simulink subsystem "ElectricalThermalSystemSSC"  (R2025a)
settings: Solver=VariableStepAuto  StartTime=0.0  StopTime=10.0  RelTol=1e-3
undefined symbols (not defined in the file): coolant_pipe_D, coolant_valve_D_ratio_max, coolant_valve_D_ratio_min, coolant_valve_displacement, EnvAirTemp, EnvGrvty, PlantThrEstCmpPwr, PlntThrChArea, PlntThrFanMaxSpd, PlntThrFanMechEff, PlntThrFanVolEff, PlntThrHeaterMaxPwr, PlntThrPipeArea, PlntThrPipeDia, PlntThrPmpMaxSpd, PlntThrRadRamEff, PlntThrRefrigAinit, PlntThrTankArea, PlntThrTankVol, PlntThrValDisp, PlntThrValDratioMax, PlntThrValDratioMin, PlntThrValSplMax, ThrmEM1, ThrmEM2, ThrmEM3, ThrmEM4
libraries: fl_lib x159, nesl_utility x69, SimscapeFluids_lib x25, autolibutils x12
(part 1 of 5)
settings Model: ModifiedByFormat=The MathWorks, Inc.  Creator=The MathWorks, Inc.  LastModifiedBy=The MathWorks, Inc.
settings SolverCC: MaxZcPerStep=1.0
settings OptimizationCC: ReuseModelBlockBuffer=off
settings DebuggingCC: UnconnectedInputMsg=warning  UnconnectedOutputMsg=warning  UnconnectedLineMsg=warning  SubsystemReferenceDiagnosticForUnitTest=warning
settings ModelReferenceCC: EnableRefExpFcnMdlSchedulingChecks=on
settings RTWCC: GPUComputeCapability=3.5  DLArmComputeVersion=19.05  LargeConstantGeneration=WriteOnlyDNNConstantsToDataFiles
settings CodeAppCC: StateflowObjectComments=on

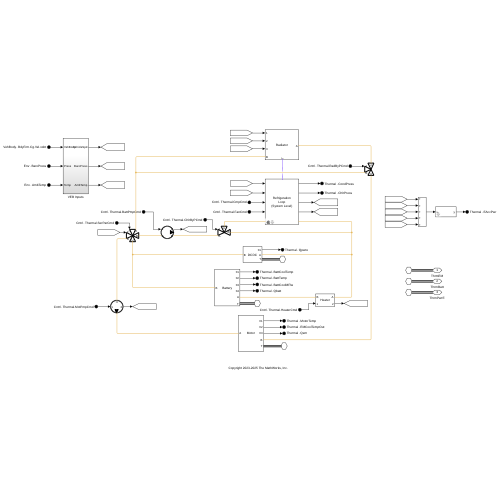
[thumbnail: Simulink's stored preview of the top-level diagram]
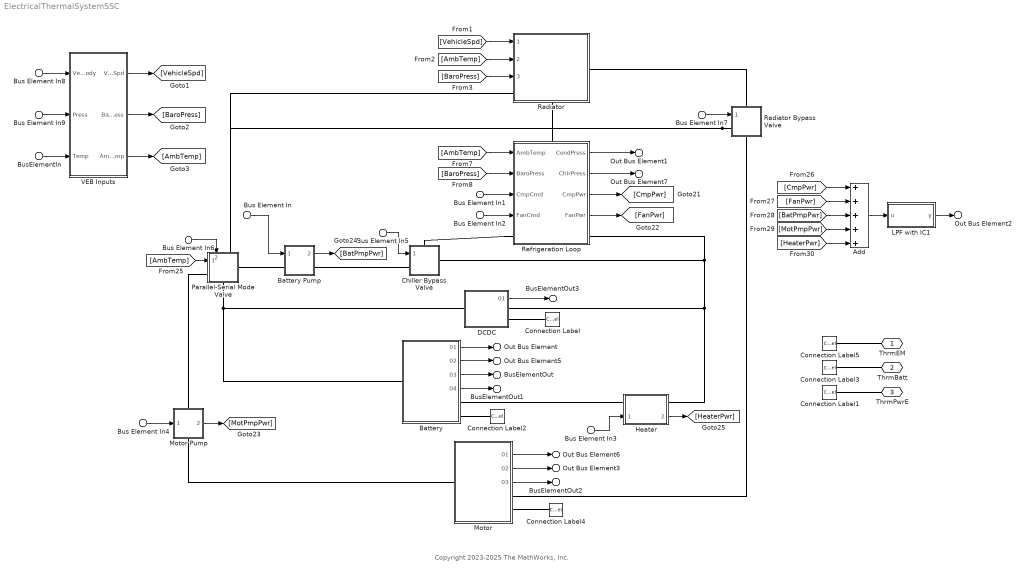
== system ElectricalThermalSystemSSC ==
  note: Copyright 2023-2025 The MathWorks, Inc.
  Bus Element In4 : Inport  PortName=Cntrl  Element=Thermal.MotPmpCmd
  Bus Element In6 : Inport  PortName=Cntrl  Element=Thermal.SerParCmd
  Bus Element In2 : Inport  PortName=Cntrl  Element=Thermal.FanCmd
  Bus Element In7 : Inport  PortName=Cntrl  Element=Thermal.RadByPCmd
  Bus Element In1 : Inport  PortName=Cntrl  Element=Thermal.CmpCmd
  Bus Element In3 : Inport  PortName=Cntrl  Element=Thermal.HeaterCmd
  Bus Element In : Inport  PortName=Cntrl  Element=Thermal.BattPmpCmd
  Bus Element In5 : Inport  PortName=Cntrl  Element=Thermal.ChlrByPCmd
  Bus Element In8 : Inport  Port=2  PortName=VehBody  Element=BdyFrm.Cg.Vel.xdot
  Bus Element In9 : Inport  Port=3  PortName=Env  Element=BaroPress
  BusElementIn : Inport  Port=3  PortName=Env  Element=AmbTemp
  Add : Sum  Inputs=+++++
  Battery : Subsystem  Tag=PublishSubsystem
      mask Display: disp(get_param(gcb, 'Name'))
  Battery Pump : Subsystem  Tag=PublishSubsystem
      mask Display:
      | plot(100*cos(linspace(0, 2*pi, 500)), 100*sin(linspace(0, 2*pi, 500)))
      | patch([100 55 55 100]-1, [0 24 -24 0], [0 0 0])
  Chiller Bypass Valve : Subsystem  Tag=PublishSubsystem
      settings: PortSchema="{\"entries\":[{\"content\":{\"sides\":[{\"content\":{\"connectorIds\":[\"In1\",\"LConn1\"]},\"type\":\"ConnectorPlacement.EquallySpacedRectSide\",\"uuid\":\"6d832dc2-b60e-40b1-a4f2-705eabcb1b94\"},{\"content\":{\"connectorIds\":[\"RConn1\"],\"side\":\"RIGHT\"},\"type\":\"ConnectorPlacement.EquallySpacedRectSide\",\"uuid\":\"14466d4b-d366-4217-9b68-7dedef557cda\"},{\"content\":{\"connectorIds\":[\"LConn2\"],\"side\":\"TOP\"},\"type\":\"ConnectorPlacement.EquallySpacedRectSide\",\"uuid\":\"a673b71e-6232-4949-9217-0d4d0fced751\"}]},\"type\":\"ConnectorPlacement.EquallySpacedConnector\",\"uuid\":\"e7c23af8-b365-4139-b104-c2b6ff749898\"}],\"packageUris\":[\"http://schema.mathworks.com/mf0/Connector/R2020b\"],\"version\":\"1.0\"}"
      mask Display:
      | color('white')
      | plot(100, 100)
      | plot(-100, -100)
      | color('black')
      | 
      | plot([0 -100 -100 0], [0 50 -50 0])
      | plot([0 100 100 0], [0 50 -50 0])
      | plot([0 50 -50 0], [0 100 100 0])
  Connection Label : ConnectionLabel  Label=ThrmPwrE
  Connection Label1 : ConnectionLabel  Label=ThrmPwrE
  Connection Label2 : ConnectionLabel  Label=ThrmBatt
  Connection Label3 : ConnectionLabel  Label=ThrmBatt
  Connection Label4 : ConnectionLabel  Label=ThrmEM
  Connection Label5 : ConnectionLabel  Label=ThrmEM
  DCDC : Subsystem  Tag=PublishSubsystem
      mask Display: disp(get_param(gcb, 'Name'))
  Heater : Subsystem  Tag=PublishSubsystem
      mask Display: disp(get_param(gcb, 'Name'))
  LPF with IC1 : Subsystem  mask{wc=10, InitCond=0, dataType=off}
      mask prompts: wc "Cutoff frequency, wc [rad/s]"; InitCond "Initial condition, InitCond [same as u]"; dataType "Enforce same input data type"
      mask TypeOptions wc: Cont LPF IC/wc
      mask TypeOptions InitCond: Initial Condition/Value
      mask TypeOptions dataType: Cont LPF IC/dataType
  Motor : Subsystem  Tag=PublishSubsystem
      mask Display: disp(get_param(gcb, 'Name'))
  Motor Pump : Subsystem  Tag=PublishSubsystem
      settings: PortSchema="{\"entries\":[{\"content\":{\"sides\":[{\"content\":{\"connectorIds\":[\"In1\"]},\"type\":\"ConnectorPlacement.EquallySpacedRectSide\",\"uuid\":\"998a9c6b-bb40-4bcc-a380-2cd5a078b990\"},{\"content\":{\"connectorIds\":[\"Out1\"],\"side\":\"RIGHT\"},\"type\":\"ConnectorPlacement.EquallySpacedRectSide\",\"uuid\":\"42ec83ef-b217-4586-a8aa-6044af8db7a9\"},{\"content\":{\"connectorIds\":[\"LConn1\"],\"side\":\"TOP\"},\"type\":\"ConnectorPlacement.EquallySpacedRectSide\",\"uuid\":\"eeac28b9-ebf8-455e-ab0a-fa40d1d96b1a\"},{\"content\":{\"connectorIds\":[\"RConn1\"],\"side\":\"BOTTOM\"},\"type\":\"ConnectorPlacement.EquallySpacedRectSide\",\"uuid\":\"020a4ae5-c25e-4792-8687-aa24bac3421e\"}]},\"type\":\"ConnectorPlacement.EquallySpacedConnector\",\"uuid\":\"d6a5444d-a0f8-4af1-be22-0f458325ee39\"}],\"packageUris\":[\"http://schema.mathworks.com/mf0/Connector/R2020b\"],\"version\":\"1.0\"}"
      mask Display:
      | plot(100*cos(linspace(0, 2*pi, 500)), 100*sin(linspace(0, 2*pi, 500)))
      | patch([0 24 -24 0], [-100 -55 -55 -100]+1, [0 0 0])
  Parallel-Serial Mode Valve : Subsystem  Tag=PublishSubsystem
      settings: PortSchema="{\"entries\":[{\"content\":{\"sides\":[{\"content\":{\"connectorIds\":[\"In1\",\"LConn1\"]},\"type\":\"ConnectorPlacement.EquallySpacedRectSide\",\"uuid\":\"0e85f4fb-5a75-439f-b35d-71055581b22a\"},{\"content\":{\"connectorIds\":[\"RConn1\"],\"side\":\"RIGHT\"},\"type\":\"ConnectorPlacement.EquallySpacedRectSide\",\"uuid\":\"a94d9cc9-a388-4b39-8755-f80106b7cded\"},{\"content\":{\"connectorIds\":[\"In2\",\"LConn2\"],\"side\":\"TOP\"},\"type\":\"ConnectorPlacement.EquallySpacedRectSide\",\"uuid\":\"13934e59-9fe7-4603-811a-b738b7f2468b\"},{\"content\":{\"connectorIds\":[\"RConn2\"],\"side\":\"BOTTOM\"},\"type\":\"ConnectorPlacement.EquallySpacedRectSide\",\"uuid\":\"987fbf53-7ea1-4dfb-bf26-1dc5077683a8\"}]},\"type\":\"ConnectorPlacement.EquallySpacedConnector\",\"uuid\":\"a78c426f-33db-4869-ab6d-8416109da949\"}],\"packageUris\":[\"http://schema.mathworks.com/mf0/Connector/R2020b\"],\"version\":\"1.0\"}"
      mask Display:
      | color('white')
      | plot(100, 100)
      | plot(-100, -100)
      | color('black')
      | 
      | plot([0 -100 -100 0], [0 50 -50 0])
      | plot([0 100 100 0], [0 50 -50 0])
      | plot([0 50 -50 0], [0 100 100 0])
      | plot([0 50 -50 0], [0 -100 -100 0])
  Radiator : Subsystem  Tag=PublishSubsystem
      settings: PortSchema="{\"entries\":[{\"content\":{\"sides\":[{\"content\":{\"connectorIds\":[\"In1\",\"In2\",\"In3\",\"LConn1\"]},\"type\":\"ConnectorPlacement.EquallySpacedRectSide\",\"uuid\":\"99a54269-bbf6-4ded-87b9-61a0201744d3\"},{\"content\":{\"connectorIds\":[\"RConn1\"],\"side\":\"RIGHT\"},\"type\":\"ConnectorPlacement.EquallySpacedRectSide\",\"uuid\":\"97272aa5-cf38-4f1e-876b-ad8adb9bd6e5\"},{\"content\":{\"side\":\"TOP\"},\"type\":\"ConnectorPlacement.EquallySpacedRectSide\",\"uuid\":\"c8198971-aa26-402f-9339-3fbe814dbf96\"},{\"content\":{\"connectorIds\":[\"RConn2\"],\"side\":\"BOTTOM\"},\"type\":\"ConnectorPlacement.EquallySpacedRectSide\",\"uuid\":\"78457e8c-40ee-463d-bbac-3ff68067e992\"}]},\"type\":\"ConnectorPlacement.EquallySpacedConnector\",\"uuid\":\"b91fbaf9-058c-42a3-b093-b88166909bf7\"}],\"packageUris\":[\"http://schema.mathworks.com/mf0/Connector/R2020b\"],\"version\":\"1.0\"}"
      mask Display: disp(get_param(gcb, 'Name'))
  Radiator Bypass Valve : Subsystem  Tag=PublishSubsystem
      settings: PortSchema="{\"entries\":[{\"content\":{\"sides\":[{\"content\":{\"connectorIds\":[\"In1\",\"LConn1\"]},\"type\":\"ConnectorPlacement.EquallySpacedRectSide\",\"uuid\":\"098431ba-fd37-427d-ab99-1fdc173a8d83\"},{\"content\":{\"side\":\"RIGHT\"},\"type\":\"ConnectorPlacement.EquallySpacedRectSide\",\"uuid\":\"bb877428-37aa-42a4-9b6a-b528d13b970d\"},{\"content\":{\"connectorIds\":[\"LConn2\"],\"side\":\"TOP\"},\"type\":\"ConnectorPlacement.EquallySpacedRectSide\",\"uuid\":\"3621d48a-02c0-4e61-a0fa-118fe0650d0a\"},{\"content\":{\"connectorIds\":[\"RConn1\"],\"side\":\"BOTTOM\"},\"type\":\"ConnectorPlacement.EquallySpacedRectSide\",\"uuid\":\"1f4bac76-5544-4b75-8f5a-621b64243fb7\"}]},\"type\":\"ConnectorPlacement.EquallySpacedConnector\",\"uuid\":\"706d2219-b4aa-4013-bee1-17248f8b2a38\"}],\"packageUris\":[\"http://schema.mathworks.com/mf0/Connector/R2020b\"],\"version\":\"1.0\"}"
      mask Display:
      | color('white')
      | plot(100, 100)
      | plot(-100, -100)
      | color('black')
      | 
      | plot([0 -100 -100 0], [0 50 -50 0])
      | plot([0 50 -50 0], [0 100 100 0])
      | plot([0 50 -50 0], [0 -100 -100 0])
  Refrigeration Loop : Subsystem  Tag=detailed cycle  Variant=on  VariantControlMode=label  VariantControl=Choice  LabelModeActiveChoice=System Level  mask{SystemChoice=System Level}
      mask prompts: SystemChoice "Choose a variant:"
      settings: PortSchema="{\"entries\":[{\"content\":{\"sides\":[{\"content\":{\"connectorIds\":[\"In1\",\"In2\",\"In3\",\"In4\",\"LConn1\"]},\"type\":\"ConnectorPlacement.EquallySpacedRectSide\",\"uuid\":\"4e244fff-03f9-4340-b01c-d55ca64bfb01\"},{\"content\":{\"connectorIds\":[\"Out1\",\"Out2\",\"Out3\",\"Out4\",\"RConn1\"],\"side\":\"RIGHT\"},\"type\":\"ConnectorPlacement.EquallySpacedRectSide\",\"uuid\":\"d8829212-1983-4dc7-b137-b6bce8b26069\"},{\"content\":{\"connectorIds\":[\"LConn2\"],\"side\":\"TOP\"},\"type\":\"ConnectorPlacement.EquallySpacedRectSide\",\"uuid\":\"473d2e24-2387-478c-ae11-a4bbaffe09fe\"}]},\"type\":\"ConnectorPlacement.EquallySpacedConnector\",\"uuid\":\"f4265e97-c303-48ef-b1e0-f8b1ed3e0934\"}],\"packageUris\":[\"http://schema.mathworks.com/mf0/Connector/R2020b\"],\"version\":\"1.0\"}"
      mask TypeOptions SystemChoice: System Level | Power Estimate
      mask Callback SystemChoice:
      | choice1 = 'System Level';
      | choice2 = 'Power Estimate';
      | if strcmp(get_param(gcb,'SystemChoice'),choice1)
      |     set_param(gcb,'LabelModeActiveChoice',choice1)
      | else
      |     set_param(gcb,'LabelModeActiveChoice',choice2)
      | end
      mask DialogControl DescTextVar Prompt: Refrigeration Loop
      mask DialogControl Container3 Prompt: Description
      mask DialogControl Control2 Prompt: This subsystem contains two variants.
      mask DialogControl Control3 Prompt: System Level: models the refrigeration cycle with Two-Phase Fluid blocks.
      mask DialogControl Control4 Prompt: Power Estimate: simple reduced order model based on coefficient of performance.
      mask Display:
      | disp([string( get_param(gcb,"name")); ...
      |       string(['(' get_param(gcb,"LabelModeActiveChoice") ')'])])
  VEB Inputs : Subsystem
  ThrmEM : PMIOPort  Side=Left
  ThrmBatt : PMIOPort  Port=2  Side=Left
  ThrmPwrE : PMIOPort  Port=3  Side=Left
  Out Bus Element3 : Outport  PortName=Thermal  Element=EMCoolTempOut
  Out Bus Element5 : Outport  PortName=Thermal  Element=BattTemp
  Out Bus Element6 : Outport  PortName=Thermal  Element=MotorTemp
  Out Bus Element1 : Outport  PortName=Thermal  Element=CondPress
  Out Bus Element2 : Outport  PortName=Thermal  Element=EAccPwr
  Out Bus Element : Outport  PortName=Thermal  Element=BattCoolTemp
  BusElementOut1 : Outport  PortName=Thermal  Element=Qbatt
  BusElementOut3 : Outport  PortName=Thermal  Element=Qpwre
  BusElementOut2 : Outport  PortName=Thermal  Element=Qem
  BusElementOut : Outport  PortName=Thermal  Element=BattCoolMFlw
  Out Bus Element7 : Outport  PortName=Thermal  Element=ChlrPress
  wires:
  BusElementIn/1 -> VEB Inputs/3(Temp)
  Bus Element In9/1 -> VEB Inputs/2(Press)
  Bus Element In8/1 -> VEB Inputs/1(VehBody)
  Motor/2(02) -> Out Bus Element3/1
  [HeaterPwr] -> Add/5
  Heater/1(2) -> [HeaterPwr]
  LPF with IC1/1(y) -> Out Bus Element2/1
  [MotPmpPwr] -> Add/4
  [BatPmpPwr] -> Add/3
  [FanPwr] -> Add/2
  [CmpPwr] -> Add/1
  Battery Pump/1(2) -> [BatPmpPwr]
  Motor Pump/1(2) -> [MotPmpPwr]
  Refrigeration Loop/4(FanPwr) -> [FanPwr]
  Refrigeration Loop/3(CmpPwr) -> [CmpPwr]
  VEB Inputs/2(BaroPress) -> [BaroPress]
  VEB Inputs/3(AmbTemp) -> [AmbTemp]
  VEB Inputs/1(VehicleSpd) -> [VehicleSpd]
  [AmbTemp] -> Parallel-Serial Mode Valve/1(1)
  Bus Element In7/1 -> Radiator Bypass Valve/1(1)
  Bus Element In6/1 -> Parallel-Serial Mode Valve/2(2)
  Bus Element In5/1 -> Chiller Bypass Valve/1(1)
  Bus Element In/1 -> Battery Pump/1(1)
  Bus Element In4/1 -> Motor Pump/1(1)
  Bus Element In3/1 -> Heater/1(1)
  Bus Element In2/1 -> Refrigeration Loop/4(FanCmd)
  Battery/2(02) -> Out Bus Element5/1
  Motor/1(01) -> Out Bus Element6/1
  Refrigeration Loop/2(ChlrPress) -> Out Bus Element7/1
  Bus Element In1/1 -> Refrigeration Loop/3(CmpCmd)
  Refrigeration Loop/1(CondPress) -> Out Bus Element1/1
  [BaroPress] -> Refrigeration Loop/2(BaroPress)
  [AmbTemp] -> Refrigeration Loop/1(AmbTemp)
  [BaroPress] -> Radiator/3(3)
  [AmbTemp] -> Radiator/2(2)
  [VehicleSpd] -> Radiator/1(1)
  Battery/1(01) -> Out Bus Element/1
  Add/1 -> LPF with IC1/1(u)
  Battery/3(03) -> BusElementOut/1
  Battery/4(04) -> BusElementOut1/1
  Motor/3(03) -> BusElementOut2/1
  DCDC/1(01) -> BusElementOut3/1
  connections:
  Radiator Bypass Valve/LConn1 -- Radiator/LConn1 -- Parallel-Serial Mode Valve/LConn2
  Battery/LConn1 -- Parallel-Serial Mode Valve/RConn2 -- DCDC/LConn1
  Heater/RConn1 -- DCDC/RConn1 -- Chiller Bypass Valve/RConn1 -- Refrigeration Loop/RConn1
  Motor Pump/LConn1 -- Parallel-Serial Mode Valve/LConn1
  Radiator/RConn2 -- Refrigeration Loop/LConn2
  Battery Pump/LConn1 -- Parallel-Serial Mode Valve/RConn1
  Refrigeration Loop/LConn1 -- Chiller Bypass Valve/LConn2
  Chiller Bypass Valve/LConn1 -- Battery Pump/RConn1
  Radiator Bypass Valve/LConn2 -- Radiator/RConn1
  Radiator Bypass Valve/RConn1 -- Motor/RConn1
  Motor Pump/RConn1 -- Motor/LConn1
  Battery/RConn1 -- Heater/LConn1
  ThrmEM/RConn1 -- Connection Label5/LConn1
  Connection Label4/LConn1 -- Motor/RConn2
  ThrmBatt/RConn1 -- Connection Label3/LConn1
  Connection Label2/LConn1 -- Battery/RConn2
  ThrmPwrE/RConn1 -- Connection Label1/LConn1
  Connection Label/LConn1 -- DCDC/RConn2

== system ElectricalThermalSystemSSC/Battery ==
  Batt Cool1 : fl_lib/Thermal/Thermal Elements/Thermal Mass  mass_type=foundation.enum.constant_variable.constant  mass=10 kg  sp_heat=PlntBattCp J/(K*kg)  mass_min=1e-6 kg  num_ports=foundation.enum.numPorts2.two  m_specify=off  m_priority=High  m=1 kg  m_nominal_specify=off  m_nominal_value=1  m_nominal_unit=kg  T_specify=on  T_priority=High  T=EnvAirTemp K  T_nominal_specify=off  T_nominal_value=1  T_nominal_unit=K  Q_specify=off  Q_priority=None  Q=0 W  Q_nominal_specify=off  Q_nominal_value=1  Q_nominal_unit=W
      settings: InternalSimscapePortConfiguration="{\"Bottom\":[],\"Left\":[{\"id\":\"M\",\"label\":\"\",\"type\":\"foundation.thermal.thermal\"}],\"Right\":[{\"id\":\"N\",\"label\":\"\",\"type\":\"foundation.thermal.thermal\"}],\"Top\":[]}"
  Coolant Jacket 1 : SimscapeFluids_lib/Thermal Liquid/Pipes & Fittings/Pipe (TL)  dynamic_compressibility=simscape.enum.onoff.on  inertia=simscape.enum.onoff.off  num_segments=1  pipe_length=PlntThrBattJacLen m  cross_section_geometry=fluids.thermal_liquid.pipes_fittings.enum.CrossSectionGeometry.Custom  pipe_diameter=0.1 m  pipe_inner_diameter=0.05 m  pipe_outer_diameter=0.1 m  pipe_width=0.1 m  pipe_height=0.1 m  pipe_major_axis=0.1 m  pipe_minor_axis=0.05 m  pipe_side=0.1 m  pipe_angle=30 deg  area=4*PlntThrChArea m^2  Dh=PlntThrChDia m  elevation_spec=foundation.enum.constant_variable.constant  elevation_gain=0 m  gravity_spec=foundation.enum.constant_variable.constant  g=EnvGrvty m/s^2  pressure_loss_spec=fluids.thermal_liquid.pipes_fittings.enum.PressureLossSpec.Haaland  local_pressure_loss_spec=fluids.thermal_liquid.pipes_fittings.enum.LocalLossSpec.AggregateLength  length_add=0 m  loss_coefficient=0.1  roughness_spec=fluids.thermal_liquid.pipes_fittings.enum.RoughnessSpec.Custom  roughness=1.5e-5 m  Re_friction_TLU=[ 400 1000 1.5e+3 3e+3 4e+3 6e+3 1e+4 2e+4 4e+4 6e+4 1e+5 1e+8 ]  friction_factor_TLU=[ 0.264 0.112 0.07099999999999999 0.0417 0.0387 0.0268 0.025 0.0232 0.0226 0.022 0.0214 0.0214 ]  Re_lam=100  Re_tur=500  shape_factor=64  mdot_nominal=[ 0.1 1 ] kg/s  p_diff_nominal=[ 0.001 0.01 ] MPa  mdot_threshold=1e-6 kg/s  wall_spec=fluids.thermal_liquid.pipes_fittings.enum.wall_spec.rigid  vol_expansion_spec=fluids.thermal_liquid.pipes_fittings.enum.VolumeExpansionSpec.Diameter  area_pressure_gain=1e-6 m^2/MPa  static_pressure_TLU=[.1, 1] MPa  area_pressure_gain_TLU=[1e-05, 1.1e-05] m^2  material_behavior_spec=fluids.thermal_liquid.pipes_fittings.enum.PipeMaterialBehavior.Linear  diameter_pressure_gain=1.2e-6 m/MPa  wall_thickness=0.05 m  elastic_modulus=69 GPa  stress_TLU=[276, 310] MPa  strain_TLU=[.004, .02]  stress_assert_action=simscape.enum.assert.action.none  stress_max=400 MPa  poisson_ratio=0.33  wall_time_constant=0.01 s  thermal_expansion=false  alpha_L_wall=24 um/(deltaK*m)  thermal_expansion_Tref=293.15 K  heat_transfer_spec=fluids.thermal_liquid.pipes_fittings.enum.HeatTransferSpec.DittusBoelter  mdot_nominal_heat=[ 0.1 1 ] kg/s  T_in_nominal=[ 293.15 293.15 ] K  T_out_nominal=[ 300 300 ] K  p_in_nominal_heat=[ 0.101325 0.101325 ] MPa  T_wall_nominal=[ 303.15 303.15 ] K  a_coeff=0.3  b_Re_power=0.8  c_Pr_power=0.33  Nu_lam=3.66  Re_Colburn_TLU=[ 100 150 1000 ]  Colburn_factor_TLU=[ 0.019 0.013 0.002 ]  Re_Nu_TLU=[ 100 150 1000 ]  Pr_Nu_TLU=[ 1 10 ]  Nu_TLU=[ 3.72 4.21; 3.75 4.44; 4.21 7.15 ]  p0_vec=EnvAbsPrs Pa  T0_vec=EnvAirTemp K  mdot0=0.1 kg/s  p_nominal=0.101325 MPa  T_nominal=293.15 K
  Flow Resistance (TL) : fl_lib/Thermal Liquid/Elements/Flow Resistance (TL)  delta_p_nominal=200 Pa  mdot_nominal=0.02 kg/s  area=PlntThrPipeArea m^2  laminar_fraction=1e-3
  Heat Flow Rate Sensor : fl_lib/Thermal/Thermal Sensors/Heat Flow Rate Sensor
  PS-Simulink Converter : nesl_utility/PS-Simulink Converter  PhysicalDomain=network_engine_domain  SubClassName=ps_output  LeftPortType=input  RightPortType=output  PseudoPeriodic=off  Frequencies=[]  VectorFormat=inherit  Unit=W  AffineConversion=off
  S1 : Subsystem
      mask Display: disp(get_param(gcb, 'Name'))
  SC1 : Subsystem
      mask Display: disp(get_param(gcb, 'Name'))
  SC2 : Subsystem
      mask Display: disp(get_param(gcb, 'Name'))
  Simscape Bus2 : SimscapeBus  HierarchyStrings=ThrmBatt1
  B : PMIOPort  Side=Left
  A : PMIOPort  Port=2  Side=Right
  T : PMIOPort  Port=3  Side=Right
  01 : Outport
  02 : Outport  Port=2
  03 : Outport  Port=3
  04 : Outport  Port=4
  wires:
  PS-Simulink Converter/1 -> 04/1
  SC2/1(01) -> 03/1
  SC1/1(BattCoolTemp) -> 01/1
  S1/1(BattTemp) -> 02/1
  connections:
  PS-Simulink Converter/LConn1 -- Heat Flow Rate Sensor/RConn1
  Heat Flow Rate Sensor/RConn2 -- S1/RConn1
  Heat Flow Rate Sensor/LConn1 -- Batt Cool1/LConn1
  T/RConn1 -- Simscape Bus2/RConn1
  Flow Resistance (TL)/RConn1 -- B/RConn1
  SC2/LConn1 -- Flow Resistance (TL)/LConn1
  SC2/RConn1 -- Coolant Jacket 1/RConn1
  A/RConn1 -- SC1/RConn1
  SC1/LConn1 -- Coolant Jacket 1/LConn1
  S1/LConn1 -- Coolant Jacket 1/LConn2
  Batt Cool1/RConn1 -- Simscape Bus2/LConn1

== system ElectricalThermalSystemSSC/Battery Pump ==
  1 : Inport
  Battery Pump : SimscapeFluids_lib/Thermal Liquid/Pumps & Motors/Fixed-Displacement Pump (TL)  loss_spec=fluids.thermal_liquid.pumps_motors.enum.LossSpec.TabulatedEfficiency  displacement=PlntThrPmpDisp l/rev  omega_nominal=0.5 * PlntThrPmpMaxSpd rpm  p_nominal=0.1 MPa  mu_nominal=0.9 cP  vol_eff_nominal=PlntThrPmpVolEff  mech_eff_nominal=PlntThrPmpMechEff  no_load_torque=0.03 N*m  p_diff_eff_TLU=[.1, 1, 2] MPa  omega_eff_TLU=[25, 50, 100, 200, 300, 400] rad/s  vol_eff_TLU=[.816, .908, .954, .977, .981, .984; .325, .663, .831, .916, .925, .946; .137, .568, .78, .892, .893, .91]  mech_eff_TLU=[.996, .996, .996, .996, .996, .996; .988, .989, .989, .989, .989, .99; .981, .981, .982, .982, .983, .984]  p_diff_loss_TLU=[.1, 1, 2] MPa  omega_loss_TLU=[25, 50, 100, 200, 300, 400] rad/s  vol_loss_TLU=[.023, .023, .023, .023, .0285, .032; .0844, .0842, .0845, .084, .1125, .108; .1079, .108, .11, .108, .1605, .18] * 1e-3 m^3/s  mech_loss_TLU=[.002, .002, .002, .002, .002, .002; .0607, .0556, .0556, .0556, .0556, .0505; .1937, .1937, .1833, .1833, .1729, .1626] N*m  vol_eff_min=1e-3  vol_eff_max=1  mech_eff_min=1e-3  mech_eff_max=1  pressure_threshold=1e-3 MPa  omega_threshold=10 rad/s  area=PlntThrPipeArea m^2  supplied_range_check=0  pump_mode_check=simscape.enum.assert.action.none  pressure_check=simscape.enum.assert.action.none  p_min_valid=0.101325 MPa
  Ideal Angular Velocity Source : fl_lib/Mechanical/Mechanical Sources/Ideal Angular Velocity Source
  Ideal Rotational Motion Sensor : fl_lib/Mechanical/Mechanical Sensors/Ideal Rotational Motion Sensor  reference=foundation.enum.MeasurementReference.difference  acceleration_port=false  velocity_port=true  position_port=true  wrap_angle=false  offset=0 rad
  Ideal Torque Sensor : fl_lib/Mechanical/Mechanical Sensors/Ideal Torque Sensor
  LPF with IC1 : Subsystem  mask{wc=0.2, InitCond=0, dataType=off}
      mask prompts: wc "Cutoff frequency, wc [rad/s]"; InitCond "Initial condition, InitCond [same as u]"; dataType "Enforce same input data type"
      mask TypeOptions wc: Cont LPF IC/wc
      mask TypeOptions InitCond: Initial Condition/Value
      mask TypeOptions dataType: Cont LPF IC/dataType
  Max Speed [rpm] : Gain  Gain=PlntThrPmpMaxSpd
  Mechanical Rotational Reference : fl_lib/Mechanical/Rotational Elements/Mechanical Rotational Reference
  Mechanical Rotational Reference1 : fl_lib/Mechanical/Rotational Elements/Mechanical Rotational Reference
  PS Product : fl_lib/Physical Signals/Functions/PS Product
  PS-Simulink Converter : nesl_utility/PS-Simulink Converter  PhysicalDomain=network_engine_domain  SubClassName=ps_output  LeftPortType=input  RightPortType=output  PseudoPeriodic=off  Frequencies=[]  VectorFormat=inherit  Unit=W  AffineConversion=off
  Simulink-PS Converter : nesl_utility/Simulink-PS Converter  PhysicalDomain=network_engine_domain  SubClassName=ps_input  LeftPortType=input  RightPortType=output  PseudoPeriodic=off  Frequencies=[]  NoiseDistribution=none  NoiseParameters=[]  Unit=rpm  AffineConversion=off  FilteringAndDerivatives=provide  SimscapeFilterOrder=1  InputFilterTimeConstant=0.001  UdotUserProvided=0
  A : PMIOPort  Side=Left
  B : PMIOPort  Port=2  Side=Right
  2 : Outport
  wires:
  LPF with IC1/1(y) -> Max Speed [rpm]/1
  1/1 -> LPF with IC1/1(u)
  Max Speed [rpm]/1 -> Simulink-PS Converter/1
  PS-Simulink Converter/1 -> 2/1
  connections:
  Simulink-PS Converter/RConn1 -- Ideal Angular Velocity Source/RConn1
  Ideal Angular Velocity Source/RConn2 -- Mechanical Rotational Reference/LConn1 -- Battery Pump/RConn2
  Battery Pump/LConn1 -- A/RConn1
  Battery Pump/LConn2 -- B/RConn1
  Mechanical Rotational Reference1/LConn1 -- Ideal Rotational Motion Sensor/RConn1
  PS Product/LConn2 -- Ideal Torque Sensor/RConn2
  PS-Simulink Converter/LConn1 -- PS Product/RConn1
  PS Product/LConn1 -- Ideal Rotational Motion Sensor/RConn2
  Ideal Torque Sensor/RConn1 -- Battery Pump/RConn1
  Ideal Torque Sensor/LConn1 -- Ideal Angular Velocity Source/LConn1 -- Ideal Rotational Motion Sensor/LConn1

== system ElectricalThermalSystemSSC/Chiller Bypass Valve ==
  1 : Inport
  Bias : Bias  Bias=-1  SaturateOnIntegerOverflow=off
  Chiller Bypass Valve : SimscapeFluids_lib/Thermal Liquid/Valves & Orifices/Directional Control Valves/3-Way Directional Valve (TL)  open_orifices_pos=fluids.thermal_liquid.valves.directional_control_valves.enum.OpenOrifices3Way.PA  open_orifices_neg=fluids.thermal_liquid.valves.directional_control_valves.enum.OpenOrifices3Way.AT  area_spec=fluids.thermal_liquid.valves.directional_control_valves.enum.area_spec.identical  valve_spec=fluids.thermal_liquid.valves.enum.orifice_spec.linear  del_S_max=PlntThrValDisp m  area_max=pi * (PlntThrValDratioMax*PlntThrPipeDia)^2 / 4 m^2  del_S_TLU=[0 0.002 0.004 0.007 0.017] m  valve_area_TLU=[1e-09, 2.0352e-07, 4.0736e-05, .00011438, .00034356] m^2  del_S_flow_TLU=[0 0.002 0.004 0.007 0.017] m  p_diff_TLU=[-.1, .3, .5, .7] MPa  vol_flow_TLU=1e-3 * [1.7e-05, 2e-05, 2.6e-05; .0035, .0045, .0053; .7, .9, 1.06; 1.96, 2.5, 3; 6, 7.7, 9.13] m^3/s  mdot_TLU=[-1e-05, 1.7e-05, 2e-05, 2.6e-05; -.002, .0035, .0045, .0053; -.4, .7, .9, 1.06; -1.13, 1.96, 2.5, 3; -3.45, 6, 7.7, 9.13] kg/s  T_ref_in=293.15 K  p_ref_in=0.101325 MPa  area_leak=pi * (PlntThrValDratioMin*PlntThrPipeDia)^2 / 4 m^2  Cd=0.7  Re_c=12  smoothing_factor=0.01  pressure_recovery=simscape.enum.onoff.on  area=pi *PlntThrPipeDia^2 / 4 m^2  S_max_PA=PlntThrValSplMax m  del_S_max_PA=coolant_valve_displacement-(coolant_valve_displacement)*(pi * (coolant_valve_D_ratio_min*coolant_pipe_D)^2 / 4)/(pi * (coolant_valve_D_ratio_max*coolant_pipe_D)^2 / 4) m  area_max_PA=pi * (coolant_valve_D_ratio_max*coolant_pipe_D)^2 / 4 m^2  del_S_TLU_PA=[0 0.002 0.004 0.007 0.017] m  valve_area_TLU_PA=[1e-09, 2.0352e-07, 4.0736e-05, .00011438, .00034356] m^2  del_S_flow_TLU_PA=[0 0.002 0.004 0.007 0.017] m  p_diff_TLU_PA=[-.1, .3, .5, .7] MPa  vol_flow_TLU_PA=1e-3 * [1.7e-05, 2e-05, 2.6e-05; .0035, .0045, .0053; .7, .9, 1.06; 1.96, 2.5, 3; 6, 7.7, 9.13] m^3/s  mdot_TLU_PA=[-1e-05, 1.7e-05, 2e-05, 2.6e-05; -.002, .0035, .0045, .0053; -.4, .7, .9, 1.06; -1.13, 1.96, 2.5, 3; -3.45, 6, 7.7, 9.13] kg/s  S_max_AT=-PlntThrValSplMax m  del_S_max_AT=coolant_valve_displacement-(coolant_valve_displacement)*(pi * (coolant_valve_D_ratio_min*coolant_pipe_D)^2 / 4)/(pi * (coolant_valve_D_ratio_max*coolant_pipe_D)^2 / 4) m  area_max_AT=pi * (coolant_valve_D_ratio_max*coolant_pipe_D)^2 / 4 m^2  del_S_TLU_AT=[0 0.002 0.004 0.007 0.017] m  valve_area_TLU_AT=[1e-09, 2.0352e-07, 4.0736e-05, .00011438, .00034356] m^2  del_S_flow_TLU_AT=[0 0.002 0.004 0.007 0.017] m  p_diff_TLU_AT=[-.1, .3, .5, .7] MPa  vol_flow_TLU_AT=1e-3 * [1.7e-05, 2e-05, 2.6e-05; .0035, .0045, .0053; .7, .9, 1.06; 1.96, 2.5, 3; 6, 7.7, 9.13] m^3/s  mdot_TLU_AT=[-1e-05, 1.7e-05, 2e-05, 2.6e-05; -.002, .0035, .0045, .0053; -.4, .7, .9, 1.06; -1.13, 1.96, 2.5, 3; -3.45, 6, 7.7, 9.13] kg/s  S_max_PT=2.5e-3 m  del_S_max_PT=0.005 m  area_max_PT=1e-4 m^2  del_S_TLU_PT=[0, .002, .004, .007, .017] m  valve_area_TLU_PT=[1e-09, 2.0352e-07, 4.0736e-05, .00011438, .00034356] m^2  del_S_flow_TLU_PT=[0, .002, .004, .007, .017] m  p_diff_TLU_PT=[.3, .5, .7] MPa  vol_flow_TLU_PT=1e-3 * [1.7e-05, 2e-05, 2.6e-05; .0035, .0045, .0053; .7, .9, 1.06; 1.96, 2.5, 3; 6, 7.7, 9.13] m^3/s  mdot_TLU_PT=[1.7e-05, 2e-05, 2.6e-05; .0035, .0045, .0053; .7, .9, 1.06; 1.96, 2.5, 3; 6, 7.7, 9.13] kg/s
      settings: InternalSimscapePortConfiguration="{\"Bottom\":[],\"Left\":[{\"id\":\"A\",\"label\":\"A\",\"type\":\"foundation.thermal_liquid.thermal_liquid\"}],\"Right\":[{\"id\":\"S\",\"label\":\"S\",\"type\":\"input\"},{\"id\":\"P\",\"label\":\"P\",\"type\":\"foundation.thermal_liquid.thermal_liquid\"},{\"id\":\"T\",\"label\":\"T\",\"type\":\"foundation.thermal_liquid.thermal_liquid\"}],\"Top\":[]}"
  Flow Resistance (TL) : fl_lib/Thermal Liquid/Elements/Flow Resistance (TL)  delta_p_nominal=0.001 MPa  mdot_nominal=0.3 kg/s  area=pi * PlntThrPipeDia^2 / 4 m^2  laminar_fraction=1e-3
  Gain : Gain  Gain=2
  LPF with IC1 : Subsystem  mask{wc=1, InitCond=0, dataType=off}
      mask prompts: wc "Cutoff frequency, wc [rad/s]"; InitCond "Initial condition, InitCond [same as u]"; dataType "Enforce same input data type"
      mask TypeOptions wc: Cont LPF IC/wc
      mask TypeOptions InitCond: Initial Condition/Value
      mask TypeOptions dataType: Cont LPF IC/dataType
  Max Valve Displacement [m] : Gain  Gain=PlntThrValDisp
  Simulink-PS Converter : nesl_utility/Simulink-PS Converter  PhysicalDomain=network_engine_domain  SubClassName=ps_input  LeftPortType=input  RightPortType=output  PseudoPeriodic=off  Frequencies=[]  NoiseDistribution=none  NoiseParameters=[]  Unit=m  AffineConversion=off  FilteringAndDerivatives=provide  SimscapeFilterOrder=1  InputFilterTimeConstant=0.001  UdotUserProvided=0
  A : PMIOPort  Side=Left
  C : PMIOPort  Port=2  Side=Left
  B : PMIOPort  Port=3  Side=Right
  wires:
  LPF with IC1/1(y) -> Gain/1
  Max Valve Displacement [m]/1 -> Simulink-PS Converter/1
  Bias/1 -> Max Valve Displacement [m]/1
  Gain/1 -> Bias/1
  1/1 -> LPF with IC1/1(u)
  connections:
  Chiller Bypass Valve/LConn1 -- A/RConn1
  Chiller Bypass Valve/RConn3 -- C/RConn1
  Chiller Bypass Valve/RConn1 -- Simulink-PS Converter/RConn1
  Chiller Bypass Valve/RConn2 -- Flow Resistance (TL)/LConn1
  Flow Resistance (TL)/RConn1 -- B/RConn1

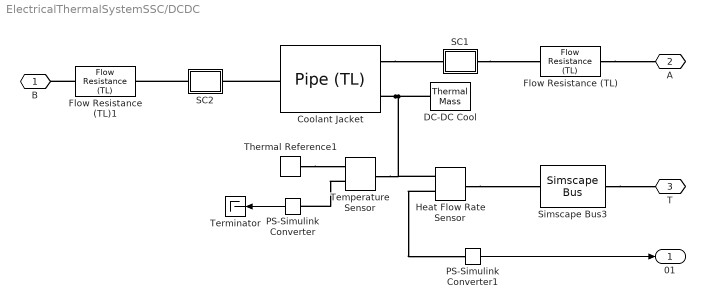
== system ElectricalThermalSystemSSC/DCDC ==
  Coolant Jacket : SimscapeFluids_lib/Thermal Liquid/Pipes & Fittings/Pipe (TL)  dynamic_compressibility=simscape.enum.onoff.on  inertia=simscape.enum.onoff.off  num_segments=1  pipe_length=PlntThrDCJacLen m  cross_section_geometry=fluids.thermal_liquid.pipes_fittings.enum.CrossSectionGeometry.Custom  pipe_diameter=0.1 m  pipe_inner_diameter=0.05 m  pipe_outer_diameter=0.1 m  pipe_width=0.1 m  pipe_height=0.1 m  pipe_major_axis=0.1 m  pipe_minor_axis=0.05 m  pipe_side=0.1 m  pipe_angle=30 deg  area=PlntThrChArea m^2  Dh=PlntThrChDia m  elevation_spec=foundation.enum.constant_variable.constant  elevation_gain=0 m  gravity_spec=foundation.enum.constant_variable.constant  g=EnvGrvty m/s^2  pressure_loss_spec=fluids.thermal_liquid.pipes_fittings.enum.PressureLossSpec.Haaland  local_pressure_loss_spec=fluids.thermal_liquid.pipes_fittings.enum.LocalLossSpec.AggregateLength  length_add=0 m  loss_coefficient=0.1  roughness_spec=fluids.thermal_liquid.pipes_fittings.enum.RoughnessSpec.Custom  roughness=1.5e-5 m  Re_friction_TLU=[ 400 1000 1.5e+3 3e+3 4e+3 6e+3 1e+4 2e+4 4e+4 6e+4 1e+5 1e+8 ]  friction_factor_TLU=[ 0.264 0.112 0.07099999999999999 0.0417 0.0387 0.0268 0.025 0.0232 0.0226 0.022 0.0214 0.0214 ]  Re_lam=100  Re_tur=500  shape_factor=64  mdot_nominal=[ 0.1 1 ] kg/s  p_diff_nominal=[ 0.001 0.01 ] MPa  mdot_threshold=1e-6 kg/s  wall_spec=fluids.thermal_liquid.pipes_fittings.enum.wall_spec.rigid  vol_expansion_spec=fluids.thermal_liquid.pipes_fittings.enum.VolumeExpansionSpec.Diameter  area_pressure_gain=1e-6 m^2/MPa  static_pressure_TLU=[.1, 1] MPa  area_pressure_gain_TLU=[1e-05, 1.1e-05] m^2  material_behavior_spec=fluids.thermal_liquid.pipes_fittings.enum.PipeMaterialBehavior.Linear  diameter_pressure_gain=1.2e-6 m/MPa  wall_thickness=0.05 m  elastic_modulus=69 GPa  stress_TLU=[276, 310] MPa  strain_TLU=[.004, .02]  stress_assert_action=simscape.enum.assert.action.none  stress_max=400 MPa  poisson_ratio=0.33  wall_time_constant=0.01 s  thermal_expansion=false  alpha_L_wall=24 um/(deltaK*m)  thermal_expansion_Tref=293.15 K  heat_transfer_spec=fluids.thermal_liquid.pipes_fittings.enum.HeatTransferSpec.DittusBoelter  mdot_nominal_heat=[ 0.1 1 ] kg/s  T_in_nominal=[ 293.15 293.15 ] K  T_out_nominal=[ 300 300 ] K  p_in_nominal_heat=[ 0.101325 0.101325 ] MPa  T_wall_nominal=[ 303.15 303.15 ] K  a_coeff=0.3  b_Re_power=0.8  c_Pr_power=0.33  Nu_lam=3.66  Re_Colburn_TLU=[ 100 150 1000 ]  Colburn_factor_TLU=[ 0.019 0.013 0.002 ]  Re_Nu_TLU=[ 100 150 1000 ]  Pr_Nu_TLU=[ 1 10 ]  Nu_TLU=[ 3.72 4.21; 3.75 4.44; 4.21 7.15 ]  p0_vec=EnvAbsPrs Pa  T0_vec=EnvAirTemp K  mdot0=0.1 kg/s  p_nominal=0.101325 MPa  T_nominal=293.15 K
  DC-DC Cool : fl_lib/Thermal/Thermal Elements/Thermal Mass  mass_type=foundation.enum.constant_variable.constant  mass=1 kg  sp_heat=PlntEMCp J/(K*kg)  mass_min=1e-6 kg  num_ports=foundation.enum.numPorts2.one  m_specify=off  m_priority=High  m=1 kg  m_nominal_specify=off  m_nominal_value=1  m_nominal_unit=kg  T_specify=on  T_priority=High  T=EnvAirTemp K  T_nominal_specify=off  T_nominal_value=1  T_nominal_unit=K  Q_specify=off  Q_priority=None  Q=0 W  Q_nominal_specify=off  Q_nominal_value=1  Q_nominal_unit=W
  Flow Resistance (TL) : fl_lib/Thermal Liquid/Elements/Flow Resistance (TL)  delta_p_nominal=2e-3 MPa  mdot_nominal=0.02 kg/s  area=PlntThrPipeArea m^2  laminar_fraction=1e-3
  Flow Resistance (TL)1 : fl_lib/Thermal Liquid/Elements/Flow Resistance (TL)  delta_p_nominal=1e-5 MPa  mdot_nominal=0.02 kg/s  area=PlntThrPipeArea m^2  laminar_fraction=1e-3
  Heat Flow Rate Sensor : fl_lib/Thermal/Thermal Sensors/Heat Flow Rate Sensor
  PS-Simulink Converter : nesl_utility/PS-Simulink Converter  PhysicalDomain=network_engine_domain  SubClassName=ps_output  LeftPortType=input  RightPortType=output  PseudoPeriodic=off  Frequencies=[]  VectorFormat=1-D array  Unit=K  AffineConversion=on
  PS-Simulink Converter1 : nesl_utility/PS-Simulink Converter  PhysicalDomain=network_engine_domain  SubClassName=ps_output  LeftPortType=input  RightPortType=output  PseudoPeriodic=off  Frequencies=[]  VectorFormat=1-D array  Unit=J/s  AffineConversion=off
  SC1 : Subsystem
      mask Display: disp(get_param(gcb, 'Name'))
  SC2 : Subsystem
      mask Display: disp(get_param(gcb, 'Name'))
  Simscape Bus3 : SimscapeBus  HierarchyStrings=ThrmPwrE1
  Temperature Sensor : fl_lib/Thermal/Thermal Sensors/Temperature Sensor  temperature_measure=foundation.enum.MeasurementReference.difference
  Terminator : Terminator
  Thermal Reference1 : fl_lib/Thermal/Thermal Elements/Thermal Reference
  B : PMIOPort  Side=Left
  A : PMIOPort  Port=2  Side=Right
  T : PMIOPort  Port=3  Side=Right
  01 : Outport
  wires:
  PS-Simulink Converter1/1 -> 01/1
  PS-Simulink Converter/1 -> Terminator/1
  connections:
  Simscape Bus3/RConn1 -- T/RConn1
  Coolant Jacket/RConn1 -- SC2/RConn1
  Coolant Jacket/LConn1 -- SC1/LConn1
  Flow Resistance (TL)1/RConn1 -- B/RConn1
  Flow Resistance (TL)/LConn1 -- A/RConn1
  SC2/LConn1 -- Flow Resistance (TL)1/LConn1
  SC1/RConn1 -- Flow Resistance (TL)/RConn1
  Temperature Sensor/RConn2 -- PS-Simulink Converter/LConn1
  Thermal Reference1/LConn1 -- Temperature Sensor/RConn1
  Coolant Jacket/LConn2 -- DC-DC Cool/LConn1 -- Heat Flow Rate Sensor/RConn2 -- Temperature Sensor/LConn1
  Heat Flow Rate Sensor/LConn1 -- Simscape Bus3/LConn1
  Heat Flow Rate Sensor/RConn1 -- PS-Simulink Converter1/LConn1

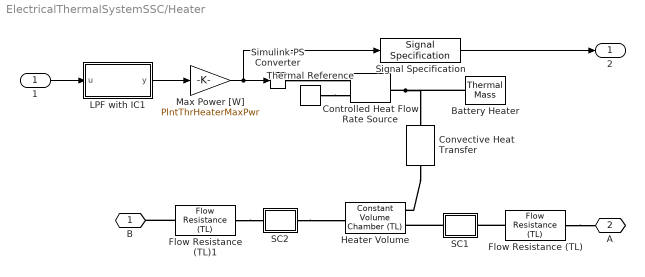
== system ElectricalThermalSystemSSC/Heater ==
  1 : Inport
  Battery Heater : fl_lib/Thermal/Thermal Elements/Thermal Mass  mass_type=foundation.enum.constant_variable.constant  mass=2 kg  sp_heat=447 J/kg/K  mass_min=1e-6 kg  num_ports=foundation.enum.numPorts2.one  m_specify=off  m_priority=High  m=1 kg  m_nominal_specify=off  m_nominal_value=1  m_nominal_unit=kg  T_specify=on  T_priority=High  T=EnvAirTemp K  T_nominal_specify=off  T_nominal_value=1  T_nominal_unit=K  Q_specify=off  Q_priority=None  Q=0 W  Q_nominal_specify=off  Q_nominal_value=1  Q_nominal_unit=W
  Controlled Heat Flow Rate Source : fl_lib/Thermal/Thermal Sources/Controlled Heat Flow Rate Source
  Convective Heat Transfer : fl_lib/Thermal/Thermal Elements/Convective Heat Transfer  thermal_type=foundation.enum.constant_variable.constant  area=PlntThrHeaterJacArea m^2  heat_tr_coeff=PlntThrHeaterCoeff W/(m^2 * K)  min_heat_tr_coeff=1e-3 W/(K*m^2)  T_specify=off  T_priority=None  T=0 K  T_nominal_specify=off  T_nominal_value=1  T_nominal_unit=K  Q_specify=off  Q_priority=None  Q=0 W  Q_nominal_specify=off  Q_nominal_value=1  Q_nominal_unit=W
  Flow Resistance (TL) : fl_lib/Thermal Liquid/Elements/Flow Resistance (TL)  delta_p_nominal=2e-4 MPa  mdot_nominal=0.15 kg/s  area=PlntThrPipeArea m^2  laminar_fraction=1e-3
  Flow Resistance (TL)1 : fl_lib/Thermal Liquid/Elements/Flow Resistance (TL)  delta_p_nominal=2e-4 MPa  mdot_nominal=0.15 kg/s  area=PlntThrPipeArea m^2  laminar_fraction=1e-3
  Heater Volume : fl_lib/Thermal Liquid/Elements/Constant Volume Chamber (TL)  volume=PlntThrHeaterJacVol m^3  num_ports=foundation.enum.num_ports.two  area_A=PlntThrPipeArea m^2  area_B=PlntThrPipeArea m^2  area_C=0.01 m^2  area_D=0.01 m^2  p_I_specify=on  p_I_priority=High  p_I=EnvAbsPrs Pa  p_I_nominal_specify=off  p_I_nominal_value=1  p_I_nominal_unit=MPa  T_I_specify=on  T_I_priority=High  T_I=EnvAirTemp K  T_I_nominal_specify=off  T_I_nominal_value=1  T_I_nominal_unit=K  u_I_specify=off  u_I_priority=None  u_I=83.90600000000001 kJ/kg  u_I_nominal_specify=off  u_I_nominal_value=1  u_I_nominal_unit=kJ/kg  rho_I_specify=off  rho_I_priority=None  rho_I=998.21 kg/m^3  rho_I_nominal_specify=off  rho_I_nominal_value=1  rho_I_nominal_unit=kg/m^3
      settings: InternalSimscapePortConfiguration="{\"Bottom\":[],\"Left\":[{\"id\":\"A\",\"label\":\"A\",\"type\":\"foundation.thermal_liquid.thermal_liquid\"},{\"id\":\"H\",\"label\":\"H\",\"type\":\"foundation.thermal.thermal\"}],\"Right\":[{\"id\":\"B\",\"label\":\"B\",\"type\":\"foundation.thermal_liquid.thermal_liquid\"}],\"Top\":[]}"
  LPF with IC1 : Subsystem  mask{wc=1, InitCond=0, dataType=off}
      mask prompts: wc "Cutoff frequency, wc [rad/s]"; InitCond "Initial condition, InitCond [same as u]"; dataType "Enforce same input data type"
      mask TypeOptions wc: Cont LPF IC/wc
      mask TypeOptions InitCond: Initial Condition/Value
      mask TypeOptions dataType: Cont LPF IC/dataType
  Max Power [W] : Gain  Gain=PlntThrHeaterMaxPwr
  SC1 : Subsystem
      mask Display: disp(get_param(gcb, 'Name'))
  SC2 : Subsystem
      mask Display: disp(get_param(gcb, 'Name'))
  Signal Specification : SignalSpecification  Unit=W
  Simulink-PS Converter : nesl_utility/Simulink-PS Converter  PhysicalDomain=network_engine_domain  SubClassName=ps_input  LeftPortType=input  RightPortType=output  PseudoPeriodic=off  Frequencies=[]  NoiseDistribution=none  NoiseParameters=[]  Unit=W  AffineConversion=off  FilteringAndDerivatives=provide  SimscapeFilterOrder=1  InputFilterTimeConstant=0.001  UdotUserProvided=0
  Thermal Reference : fl_lib/Thermal/Thermal Elements/Thermal Reference
  B : PMIOPort  Side=Left
  A : PMIOPort  Port=2  Side=Right
  2 : Outport
  wires:
  Signal Specification/1 -> 2/1
  1/1 -> LPF with IC1/1(u)
  LPF with IC1/1(y) -> Max Power [W]/1
  Max Power [W]/1 -> Simulink-PS Converter/1, Signal Specification/1
  connections:
  Flow Resistance (TL)1/LConn1 -- SC2/LConn1
  Flow Resistance (TL)/RConn1 -- SC1/RConn1
  Convective Heat Transfer/RConn1 -- Heater Volume/LConn2
  SC2/RConn1 -- Heater Volume/RConn1
  Flow Resistance (TL)/LConn1 -- A/RConn1
  SC1/LConn1 -- Heater Volume/LConn1
  Thermal Reference/LConn1 -- Controlled Heat Flow Rate Source/RConn2
  Simulink-PS Converter/RConn1 -- Controlled Heat Flow Rate Source/RConn1
  Controlled Heat Flow Rate Source/LConn1 -- Convective Heat Transfer/LConn1 -- Battery Heater/LConn1
  Flow Resistance (TL)1/RConn1 -- B/RConn1

== system ElectricalThermalSystemSSC/LPF with IC1 ==
  u : Inport
  Cont LPF IC : autolibutils/Cont LPF IC  wc=wc  aMode=1  dataType=off
  Initial Condition : Constant  Value=InitCond  SampleTime=-1
  y : Outport
  wires:
  Cont LPF IC/1 -> y/1
  u/1 -> Cont LPF IC/1
  Initial Condition/1 -> Cont LPF IC/2

== system ElectricalThermalSystemSSC/Motor ==
  Cooling Assembly : Subsystem  Variant=on  VariantControl=Cooling Assembly  EmptyChoice=on
  PS-Simulink Converter : nesl_utility/PS-Simulink Converter  PhysicalDomain=network_engine_domain  SubClassName=ps_output  LeftPortType=input  RightPortType=output  PseudoPeriodic=off  Frequencies=[]  VectorFormat=inherit  Unit=K  AffineConversion=on
  Pressure & Temperature Sensor (TL) : fl_lib/Thermal Liquid/Sensors/Pressure & Temperature Sensor (TL)  reference=foundation.enum.MeasurementReference.absolute  pressure=false  pressure_spec=foundation.enum.PressureMeasementSpec.Absolute  temperature=true
      settings: InternalSimscapePortConfiguration="{\"Bottom\":[{\"id\":\"T\",\"label\":\"T\",\"type\":\"output\"}],\"Left\":[{\"id\":\"A\",\"label\":\"A\",\"type\":\"foundation.thermal_liquid.thermal_liquid\"}],\"Right\":[],\"Top\":[]}"
  Simscape Bus1 : SimscapeBus  HierarchyStrings=ThrmEM4;ThrmEM3;ThrmEM2;ThrmEM1
  A : PMIOPort  Side=Left
  B : PMIOPort  Port=2  Side=Right
  T : PMIOPort  Port=3  Side=Right
  01 : Outport
  02 : Outport  Port=2
  03 : Outport  Port=3
  wires:
  Cooling Assembly/2(Qem) -> 03/1
  Cooling Assembly/1(EMTemp) -> 01/1
  PS-Simulink Converter/1 -> 02/1
  connections:
  A/RConn1 -- Cooling Assembly/LConn1
  T/RConn1 -- Simscape Bus1/RConn1
  Cooling Assembly/RConn1 -- B/RConn1 -- Pressure & Temperature Sensor (TL)/LConn1
  Simscape Bus1/LConn4 -- Cooling Assembly/RConn5
  Simscape Bus1/LConn3 -- Cooling Assembly/RConn4
  Simscape Bus1/LConn2 -- Cooling Assembly/RConn3
  Simscape Bus1/LConn1 -- Cooling Assembly/RConn2
  PS-Simulink Converter/LConn1 -- Pressure & Temperature Sensor (TL)/RConn1

== system ElectricalThermalSystemSSC/Motor Pump ==
  1 : Inport
  Ideal Angular Velocity Source : fl_lib/Mechanical/Mechanical Sources/Ideal Angular Velocity Source
  Ideal Rotational Motion Sensor : fl_lib/Mechanical/Mechanical Sensors/Ideal Rotational Motion Sensor  reference=foundation.enum.MeasurementReference.difference  acceleration_port=false  velocity_port=true  position_port=true  wrap_angle=false  offset=0 rad
  Ideal Torque Sensor : fl_lib/Mechanical/Mechanical Sensors/Ideal Torque Sensor
  LPF with IC1 : Subsystem  mask{wc=0.2, InitCond=0, dataType=off}
      mask prompts: wc "Cutoff frequency, wc [rad/s]"; InitCond "Initial condition, InitCond [same as u]"; dataType "Enforce same input data type"
      mask TypeOptions wc: Cont LPF IC/wc
      mask TypeOptions InitCond: Initial Condition/Value
      mask TypeOptions dataType: Cont LPF IC/dataType
  Max Speed [rpm] : Gain  Gain=PlntThrPmpMaxSpd
  Mechanical Rotational Reference : fl_lib/Mechanical/Rotational Elements/Mechanical Rotational Reference
  Mechanical Rotational Reference1 : fl_lib/Mechanical/Rotational Elements/Mechanical Rotational Reference
  Motor Pump : SimscapeFluids_lib/Thermal Liquid/Pumps & Motors/Fixed-Displacement Pump (TL)  loss_spec=fluids.thermal_liquid.pumps_motors.enum.LossSpec.TabulatedEfficiency  displacement=PlntThrPmpDisp l/rev  omega_nominal=0.5 * PlntThrPmpMaxSpd rpm  p_nominal=0.1 MPa  mu_nominal=0.9 cP  vol_eff_nominal=PlntThrPmpVolEff  mech_eff_nominal=PlntThrPmpMechEff  no_load_torque=0.03 N*m  p_diff_eff_TLU=[.1, 1, 2] MPa  omega_eff_TLU=[25, 50, 100, 200, 300, 400] rad/s  vol_eff_TLU=[.816, .908, .954, .977, .981, .984; .325, .663, .831, .916, .925, .946; .137, .568, .78, .892, .893, .91]  mech_eff_TLU=[.996, .996, .996, .996, .996, .996; .988, .989, .989, .989, .989, .99; .981, .981, .982, .982, .983, .984]  p_diff_loss_TLU=[.1, 1, 2] MPa  omega_loss_TLU=[25, 50, 100, 200, 300, 400] rad/s  vol_loss_TLU=[.023, .023, .023, .023, .0285, .032; .0844, .0842, .0845, .084, .1125, .108; .1079, .108, .11, .108, .1605, .18] * 1e-3 m^3/s  mech_loss_TLU=[.002, .002, .002, .002, .002, .002; .0607, .0556, .0556, .0556, .0556, .0505; .1937, .1937, .1833, .1833, .1729, .1626] N*m  vol_eff_min=1e-3  vol_eff_max=1  mech_eff_min=1e-3  mech_eff_max=1  pressure_threshold=1e-3 MPa  omega_threshold=10 rad/s  area=PlntThrPipeArea m^2  supplied_range_check=0  pump_mode_check=simscape.enum.assert.action.none  pressure_check=simscape.enum.assert.action.none  p_min_valid=0.101325 MPa
  PS Product : fl_lib/Physical Signals/Functions/PS Product
  PS-Simulink Converter : nesl_utility/PS-Simulink Converter  PhysicalDomain=network_engine_domain  SubClassName=ps_output  LeftPortType=input  RightPortType=output  PseudoPeriodic=off  Frequencies=[]  VectorFormat=inherit  Unit=W  AffineConversion=off
  Simulink-PS Converter : nesl_utility/Simulink-PS Converter  PhysicalDomain=network_engine_domain  SubClassName=ps_input  LeftPortType=input  RightPortType=output  PseudoPeriodic=off  Frequencies=[]  NoiseDistribution=none  NoiseParameters=[]  Unit=rpm  AffineConversion=off  FilteringAndDerivatives=provide  SimscapeFilterOrder=1  InputFilterTimeConstant=0.001  UdotUserProvided=0
  A : PMIOPort  Side=Left
  B : PMIOPort  Port=2  Side=Right
  2 : Outport
  wires:
  1/1 -> LPF with IC1/1(u)
  LPF with IC1/1(y) -> Max Speed [rpm]/1
  Max Speed [rpm]/1 -> Simulink-PS Converter/1
  PS-Simulink Converter/1 -> 2/1
  connections:
  Simulink-PS Converter/RConn1 -- Ideal Angular Velocity Source/RConn1
  Mechanical Rotational Reference/LConn1 -- Motor Pump/RConn2 -- Ideal Angular Velocity Source/RConn2
  Motor Pump/LConn1 -- A/RConn1
  Motor Pump/LConn2 -- B/RConn1
  PS Product/LConn2 -- Ideal Torque Sensor/RConn2
  PS Product/LConn1 -- Ideal Rotational Motion Sensor/RConn2
  Mechanical Rotational Reference1/LConn1 -- Ideal Rotational Motion Sensor/RConn1
  PS Product/RConn1 -- PS-Simulink Converter/LConn1
  Motor Pump/RConn1 -- Ideal Torque Sensor/RConn1
  Ideal Torque Sensor/LConn1 -- Ideal Angular Velocity Source/LConn1 -- Ideal Rotational Motion Sensor/LConn1
